simulink model "untitled2"  (R2015b)
settings: Solver=VariableStepAuto  StartTime=0.0  StopTime=10.0  RelTol=1e-3
values from neighbouring files (symbols this model uses):
  D = img(max(r2+(c2-1)*sx,1))    [IntegralImage_BoxIntegral_mine.m]
undefined symbols (not defined in the file or in its folder): IsPositionTracked, IsSkeletonTracked, JointDepthIndices, JointImageIndices, JointTrackingState, JointWorldCoordinates, none, PositionDepthIndices, PositionImageIndices, PositionWorldCoordinates, SegmentationData, SkeletonTrackingID, videoinput
libraries: imaqlib x1
(part 5 of 5)

== matlab function untitled2/extract_features ==
  data: u input; y output
function y = fcn(u)
y=getSURF_surf(u);
%y=linspace(1,10);
